simulink model "Appl_DrMemory_CtrlModel"  (R2018b)
settings: configuration reference "CodeConfig_10_ms" (kept outside this file)
undefined symbols (not defined in the file): CAL_DrMem_100MS, CAL_DrMem_90MS, D_DRMEM_SPEED_5, D_ToleranceDistance, FALSE, TRUE
libraries: DareLib x92, simulink x1
(part 1 of 3)
settings Model: Creator=Administrator  LastModifiedBy=Administrator
settings ConfigSetRef: SourceLocation=Base Workspace

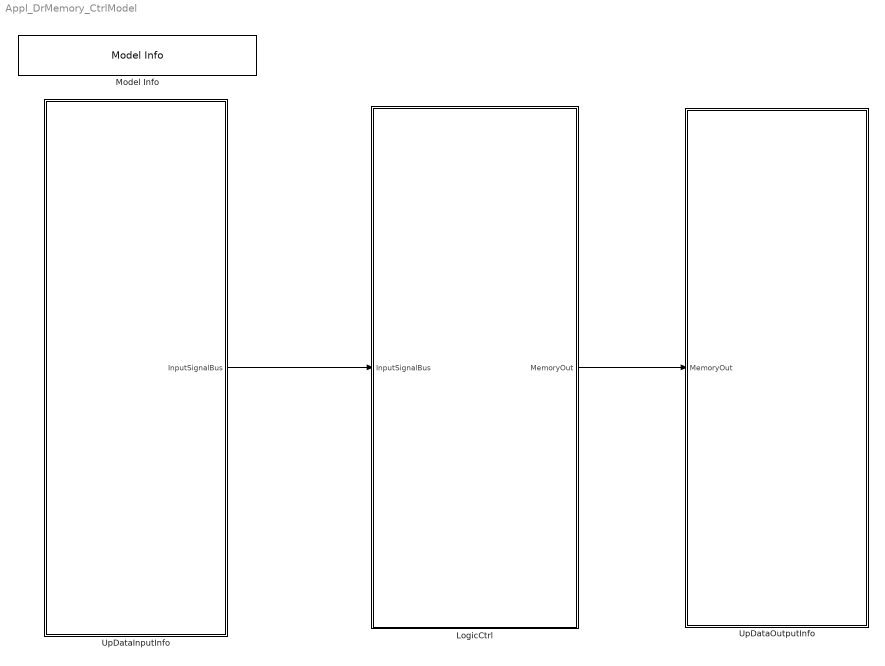
== system Appl_DrMemory_CtrlModel ==
  LogicCtrl : Subsystem  Priority=2  TreatAsAtomicUnit=on
      settings: RTWSystemCode=Nonreusable function  RTWFcnNameOpts=Use subsystem name
  Model Info : simulink/Model-Wide Utilities/Model Info  Frame=on  DisplayStringWithTags=Version：%<ModelVersion>  HorizontalTextAlignment=Center  LeftAlignmentValue=0.5
  UpDataInputInfo : Subsystem  Priority=1  TreatAsAtomicUnit=on
      settings: RTWSystemCode=Nonreusable function  RTWFcnNameOpts=Use subsystem name
  UpDataOutputInfo : Subsystem  Priority=3  TreatAsAtomicUnit=on
      settings: RTWSystemCode=Nonreusable function  RTWFcnNameOpts=Use subsystem name
  wires:
  LogicCtrl/1(MemoryOut) -> UpDataOutputInfo/1(MemoryOut)
  UpDataInputInfo/1(InputSignalBus) -> LogicCtrl/1(InputSignalBus)

== system Appl_DrMemory_CtrlModel/LogicCtrl ==
  InputSignalBus : Inport
  Bus Selector : BusSelector  OutputSignals=SpeedLessThan5_Flag,SeatMemBtn,CallMem,MemorySetPrecondition,MemoryRemindPrecondition,Rte_SignalBus.DrMem_HeightHallPosi,Rte_SignalBus.DrMem_LengthHallPosi,Rte_SignalBus.DrMem_BackHallPosi,Rte_SignalBus.DrMem_FrontHallPosi,Rte_SignalBus.DrMem_HeightAutoRunFlag,Rte_SignalBus.DrMem_LengthAutoRunFlag,Rte_SignalBus.DrMem_BackAutoRunFlag,Rte_SignalBus.DrMem_FrontAutoRunFlag,Rte_SignalBus.DrMem_AdjustEnable,Rte_SignalBus.DrMem_FLSeatPosMsg,Rte_SignalBus.DrMem_CurrentMoveType,Rte_SignalBus.DrMem_GetRecoverDefaultFlag,Rte_SignalBus.DrMem_HeightLockFault,Rte_SignalBus.DrMem_LengthLockFault,Rte_SignalBus.DrMem_BackLockFault,Rte_SignalBus.DrMem_FrontLockFault
  LocalAdjustCtrl : Subsystem  Description=加热逻辑处理
      settings: AttributesFormatString=%<Description>
  MainVent_OutputLvlSts : BusCreator  Inputs=14
  MemoryOut : Outport
  wires:
  InputSignalBus/1 -> Bus Selector/1  "InputSignalBus"
  MainVent_OutputLvlSts/1 -> MemoryOut/1  "MemoryOut"
  Bus Selector/2 -> LocalAdjustCtrl/1(SeatMemBtn)  "<SeatMemBtn>"
  Bus Selector/3 -> LocalAdjustCtrl/2(CallMem)  "<CallMem>"
  Bus Selector/4 -> LocalAdjustCtrl/3(MemorySetPrecondition)  "<MemorySetPrecondition>"
  Bus Selector/5 -> LocalAdjustCtrl/4(MemoryRemindPrecondition)  "<MemoryRemindPrecondition>"
  Bus Selector/6 -> LocalAdjustCtrl/5(DrMem_HeightHallPosi)  "<DrMem_HeightHallPosi>"
  Bus Selector/7 -> LocalAdjustCtrl/6(DrMem_LengthHallPosi)  "<DrMem_LengthHallPosi>"
  Bus Selector/8 -> LocalAdjustCtrl/7(DrMem_BackHallPosi)  "<DrMem_BackHallPosi>"
  Bus Selector/9 -> LocalAdjustCtrl/8(DrMem_FrontHallPosi)  "<DrMem_FrontHallPosi>"
  Bus Selector/10 -> LocalAdjustCtrl/9(DrMem_HeightAutoRunFlag)  "<DrMem_HeightAutoRunFlag>"
  Bus Selector/11 -> LocalAdjustCtrl/10(DrMem_LengthAutoRunFlag)  "<DrMem_LengthAutoRunFlag>"
  Bus Selector/12 -> LocalAdjustCtrl/11(DrMem_BackAutoRunFlag)  "<DrMem_BackAutoRunFlag>"
  Bus Selector/13 -> LocalAdjustCtrl/12(DrMem_FrontAutoRunFlag)  "<DrMem_FrontAutoRunFlag>"
  Bus Selector/14 -> LocalAdjustCtrl/13(DrMem_AdjustEnable)  "<DrMem_AdjustEnable>"
  Bus Selector/15 -> LocalAdjustCtrl/14(DrMem_FLSeatPosMsg)  "<DrMem_FLSeatPosMsg>"
  Bus Selector/16 -> LocalAdjustCtrl/15(DrMem_CurrentMoveType)  "<DrMem_CurrentMoveType>"
  Bus Selector/17 -> LocalAdjustCtrl/16(DrMem_GetRecoverDefaultFlag)  "<DrMem_GetRecoverDefaultFlag>"
  Bus Selector/18 -> LocalAdjustCtrl/17(DrMem_HeightLockFault)  "<DrMem_HeightLockFault>"
  Bus Selector/19 -> LocalAdjustCtrl/18(DrMem_LengthLockFault)  "<DrMem_LengthLockFault>"
  Bus Selector/20 -> LocalAdjustCtrl/19(DrMem_BackLockFault)  "<DrMem_BackLockFault>"
  Bus Selector/21 -> LocalAdjustCtrl/20(DrMem_FrontLockFault)  "<DrMem_FrontLockFault>"
  LocalAdjustCtrl/1(FLSeatMemSetSts) -> MainVent_OutputLvlSts/2
  LocalAdjustCtrl/2(MemSetStopReason) -> MainVent_OutputLvlSts/3
  LocalAdjustCtrl/3(FLSeatPosMsg) -> MainVent_OutputLvlSts/4
  LocalAdjustCtrl/4(SeatMemoryValidReq) -> MainVent_OutputLvlSts/5
  LocalAdjustCtrl/5(SeatHeightPosiReq) -> MainVent_OutputLvlSts/6
  LocalAdjustCtrl/6(SeatLengthPosiReq) -> MainVent_OutputLvlSts/7
  LocalAdjustCtrl/7(SeatBackPosiReq) -> MainVent_OutputLvlSts/8
  LocalAdjustCtrl/8(SeatFrontPosiReq) -> MainVent_OutputLvlSts/9
  LocalAdjustCtrl/9(MemCallStopReason) -> MainVent_OutputLvlSts/10
  LocalAdjustCtrl/10(SeatMem1StsFb) -> MainVent_OutputLvlSts/11
  LocalAdjustCtrl/11(SeatMem2StsFb) -> MainVent_OutputLvlSts/12
  LocalAdjustCtrl/12(SeatMem3StsFb) -> MainVent_OutputLvlSts/13
  LocalAdjustCtrl/13(PreMemRemindStop) -> MainVent_OutputLvlSts/14
  Bus Selector/1 -> MainVent_OutputLvlSts/1  "<SpeedLessThan5_Flag>"

== system Appl_DrMemory_CtrlModel/UpDataInputInfo ==
  InputSignalProcess : Subsystem  Description=数据处理
      settings: AttributesFormatString=%<Description>  RTWSystemCode=Nonreusable function  RTWFcnNameOpts=Use subsystem name
  RTE : Subsystem  Description=接口自动生成  TreatAsAtomicUnit=on
      settings: AttributesFormatString=%<Description>  RTWSystemCode=Nonreusable function  RTWFcnNameOpts=Use subsystem name
  InputSignalBus : Outport
  wires:
  RTE/1(RTE_Signal) -> InputSignalProcess/1(Rte_SignalBus)
  InputSignalProcess/1(InputSignalBus) -> InputSignalBus/1

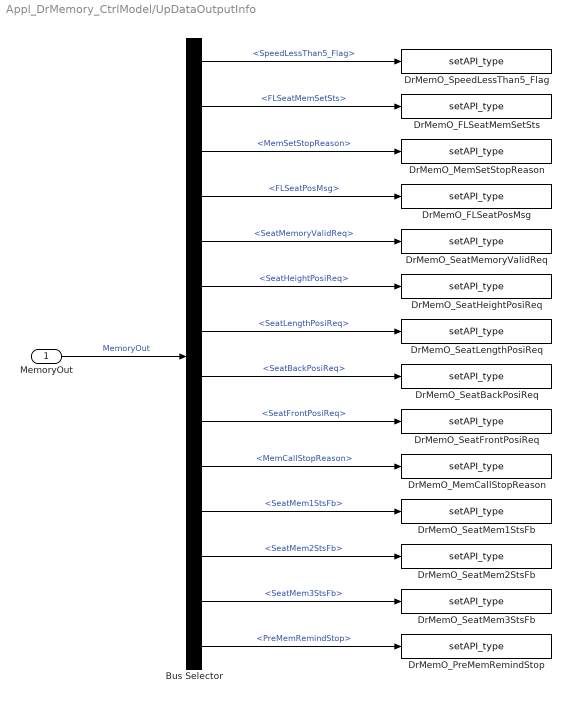
== system Appl_DrMemory_CtrlModel/UpDataOutputInfo ==
  MemoryOut : Inport
  Bus Selector : BusSelector  OutputSignals=SpeedLessThan5_Flag,FLSeatMemSetSts,MemSetStopReason,FLSeatPosMsg,SeatMemoryValidReq,SeatHeightPosiReq,SeatLengthPosiReq,SeatBackPosiReq,SeatFrontPosiReq,MemCallStopReason,SeatMem1StsFb,SeatMem2StsFb,SeatMem3StsFb,PreMemRemindStop
  DrMemO_FLSeatMemSetSts : DareLib/Dare/setAPI_type  g_funcname=CanTx_0x3B2_DSM_FLSeatMemStsAndMsg  g_param=""  g_type=uint8  g_enum=enMemSetFb  g_size=-1
      settings: AttributesFormatString=%<g_funcname>  SourceProductName=Dare Library
  DrMemO_FLSeatPosMsg : DareLib/Dare/setAPI_type  g_funcname=CanTx_0x3B2_DSM_FLSeatPosMsg  g_param=""  g_type=uint8  g_size=-1
      settings: AttributesFormatString=%<g_funcname>  SourceProductName=Dare Library
  DrMemO_MemCallStopReason : DareLib/Dare/setAPI_type  g_funcname=Rte_SetVfb_MemCallStopReason  g_param=""  g_type=uint8  g_enum=enMemStopCause  g_size=-1
      settings: AttributesFormatString=%<g_funcname>  SourceProductName=Dare Library
  DrMemO_MemSetStopReason : DareLib/Dare/setAPI_type  g_funcname=Rte_SetVfb_MemSetStopReason  g_param=""  g_type=uint8  g_enum=enMemStopCause  g_size=-1
      settings: AttributesFormatString=%<g_funcname>  SourceProductName=Dare Library
  DrMemO_PreMemRemindStop : DareLib/Dare/setAPI_type  g_funcname=Rte_SetVfb_PreMemRemindStop  g_param=""  g_type=uint8  g_enum=enMemStopCause  g_size=-1
      settings: AttributesFormatString=%<g_funcname>  SourceProductName=Dare Library
  DrMemO_SeatBackPosiReq : DareLib/Dare/setAPI_type  g_funcname=Rte_SetVfb_DrMemBackReqPosi  g_param=""  g_type=uint16  g_size=-1
      settings: AttributesFormatString=%<g_funcname>  SourceProductName=Dare Library
  DrMemO_SeatFrontPosiReq : DareLib/Dare/setAPI_type  g_funcname=Rte_SetVfb_DrMemFrontReqPosi  g_param=""  g_type=uint16  g_size=-1
      settings: AttributesFormatString=%<g_funcname>  SourceProductName=Dare Library
  DrMemO_SeatHeightPosiReq : DareLib/Dare/setAPI_type  g_funcname=Rte_SetVfb_DrMemHeightReqPosi  g_param=""  g_type=uint16  g_size=-1
      settings: AttributesFormatString=%<g_funcname>  SourceProductName=Dare Library
  DrMemO_SeatLengthPosiReq : DareLib/Dare/setAPI_type  g_funcname=Rte_SetVfb_DrMemLengthReqPosi  g_param=""  g_type=uint16  g_size=-1
      settings: AttributesFormatString=%<g_funcname>  SourceProductName=Dare Library
  DrMemO_SeatMem1StsFb : DareLib/Dare/setAPI_type  g_funcname=CanTx_0x3B2_DSM1_FLSeatMem1Sts  g_param=""  g_type=uint8  g_enum=enMemCallFb  g_size=-1
      settings: AttributesFormatString=%<g_funcname>  SourceProductName=Dare Library
  DrMemO_SeatMem2StsFb : DareLib/Dare/setAPI_type  g_funcname=CanTx_0x3B2_DSM2_FLSeatMem2Sts  g_param=""  g_type=uint8  g_enum=enMemCallFb  g_size=-1
      settings: AttributesFormatString=%<g_funcname>  SourceProductName=Dare Library
  DrMemO_SeatMem3StsFb : DareLib/Dare/setAPI_type  g_funcname=CanTx_0x3B2_DSM3_FLSeatMem3Sts  g_param=""  g_type=uint8  g_enum=enMemCallFb  g_size=-1
      settings: AttributesFormatString=%<g_funcname>  SourceProductName=Dare Library
  DrMemO_SeatMemoryValidReq : DareLib/Dare/setAPI_type  g_funcname=Rte_SetVfb_SeatMemoryValidReq  g_param=""  g_type=uint8  g_size=-1
      settings: AttributesFormatString=%<g_funcname>  SourceProductName=Dare Library
  DrMemO_SpeedLessThan5_Flag : DareLib/Dare/setAPI_type  g_funcname=Rte_SetVfb_SpeedLessThan5_Flag  g_param=""  g_type=uint8  g_size=-1
      settings: AttributesFormatString=%<g_funcname>  SourceProductName=Dare Library
  wires:
  MemoryOut/1 -> Bus Selector/1  "MemoryOut"
  Bus Selector/1 -> DrMemO_SpeedLessThan5_Flag/1  "<SpeedLessThan5_Flag>"
  Bus Selector/2 -> DrMemO_FLSeatMemSetSts/1  "<FLSeatMemSetSts>"
  Bus Selector/3 -> DrMemO_MemSetStopReason/1  "<MemSetStopReason>"
  Bus Selector/4 -> DrMemO_FLSeatPosMsg/1  "<FLSeatPosMsg>"
  Bus Selector/5 -> DrMemO_SeatMemoryValidReq/1  "<SeatMemoryValidReq>"
  Bus Selector/6 -> DrMemO_SeatHeightPosiReq/1  "<SeatHeightPosiReq>"
  Bus Selector/7 -> DrMemO_SeatLengthPosiReq/1  "<SeatLengthPosiReq>"
  Bus Selector/8 -> DrMemO_SeatBackPosiReq/1  "<SeatBackPosiReq>"
  Bus Selector/9 -> DrMemO_SeatFrontPosiReq/1  "<SeatFrontPosiReq>"
  Bus Selector/10 -> DrMemO_MemCallStopReason/1  "<MemCallStopReason>"
  Bus Selector/11 -> DrMemO_SeatMem1StsFb/1  "<SeatMem1StsFb>"
  Bus Selector/12 -> DrMemO_SeatMem2StsFb/1  "<SeatMem2StsFb>"
  Bus Selector/13 -> DrMemO_SeatMem3StsFb/1  "<SeatMem3StsFb>"
  Bus Selector/14 -> DrMemO_PreMemRemindStop/1  "<PreMemRemindStop>"

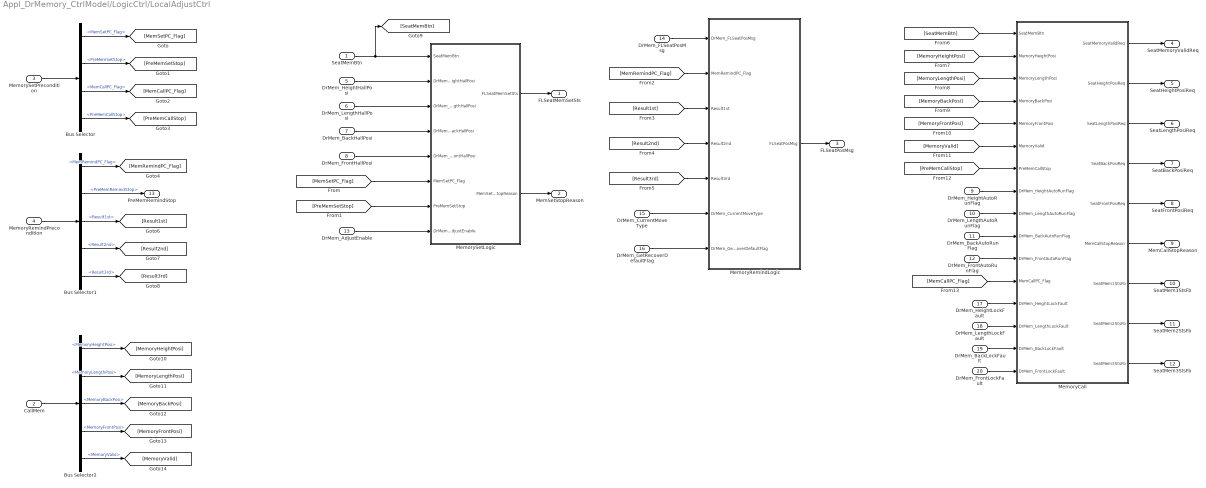
== system Appl_DrMemory_CtrlModel/LogicCtrl/LocalAdjustCtrl ==
  SeatMemBtn : Inport
  CallMem : Inport  Port=2
  MemorySetPrecondition : Inport  Port=3
  MemoryRemindPrecondition : Inport  Port=4
  DrMem_HeightHallPosi : Inport  Port=5
  DrMem_LengthHallPosi : Inport  Port=6
  DrMem_BackHallPosi : Inport  Port=7
  DrMem_FrontHallPosi : Inport  Port=8
  DrMem_HeightAutoRunFlag : Inport  Port=9
  DrMem_LengthAutoRunFlag : Inport  Port=10
  DrMem_BackAutoRunFlag : Inport  Port=11
  DrMem_FrontAutoRunFlag : Inport  Port=12
  DrMem_AdjustEnable : Inport  Port=13
  DrMem_FLSeatPosMsg : Inport  Port=14
  DrMem_CurrentMoveType : Inport  Port=15
  DrMem_GetRecoverDefaultFlag : Inport  Port=16
  DrMem_HeightLockFault : Inport  Port=17
  DrMem_LengthLockFault : Inport  Port=18
  DrMem_BackLockFault : Inport  Port=19
  DrMem_FrontLockFault : Inport  Port=20
  Bus Selector : BusSelector  OutputSignals=MemSetPC_Flag,PreMemSetStop,MemCallPC_Flag,PreMemCallStop
  Bus Selector1 : BusSelector  OutputSignals=MemRemindPC_Flag,PreMemRemindStop,Result1st,Result2nd,Result3rd
  Bus Selector2 : BusSelector  OutputSignals=MemoryHeightPosi,MemoryLengthPosi,MemoryBackPosi,MemoryFrontPosi,MemoryValid
  MemoryCall : Stateflow chart  TreatAsAtomicUnit=on
  MemoryRemindLogic : Stateflow chart  TreatAsAtomicUnit=on
  MemorySetLogic : Stateflow chart  TreatAsAtomicUnit=on
  FLSeatMemSetSts : Outport
  MemSetStopReason : Outport  Port=2
  FLSeatPosMsg : Outport  Port=3
  SeatMemoryValidReq : Outport  Port=4
  SeatHeightPosiReq : Outport  Port=5
  SeatLengthPosiReq : Outport  Port=6
  SeatBackPosiReq : Outport  Port=7
  SeatFrontPosiReq : Outport  Port=8
  MemCallStopReason : Outport  Port=9
  SeatMem1StsFb : Outport  Port=10
  SeatMem2StsFb : Outport  Port=11
  SeatMem3StsFb : Outport  Port=12
  PreMemRemindStop : Outport  Port=13
  wires:
  SeatMemBtn/1 -> [SeatMemBtn], MemorySetLogic/1(SeatMemBtn)
  DrMem_HeightHallPosi/1 -> MemorySetLogic/2(DrMem_HeightHallPosi)
  DrMem_LengthHallPosi/1 -> MemorySetLogic/3(DrMem_LengthHallPosi)
  DrMem_BackHallPosi/1 -> MemorySetLogic/4(DrMem_BackHallPosi)
  DrMem_FrontHallPosi/1 -> MemorySetLogic/5(DrMem_FrontHallPosi)
  MemorySetPrecondition/1 -> Bus Selector/1
  Bus Selector/1 -> [MemSetPC_Flag]  "<MemSetPC_Flag>"
  Bus Selector/2 -> [PreMemSetStop]  "<PreMemSetStop>"
  Bus Selector/3 -> [MemCallPC_Flag]  "<MemCallPC_Flag>"
  Bus Selector/4 -> [PreMemCallStop]  "<PreMemCallStop>"
  [MemSetPC_Flag] -> MemorySetLogic/6(MemSetPC_Flag)
  [PreMemSetStop] -> MemorySetLogic/7(PreMemSetStop)
  DrMem_AdjustEnable/1 -> MemorySetLogic/8(DrMem_AdjustEnable)
  MemoryRemindPrecondition/1 -> Bus Selector1/1
  Bus Selector1/4 -> [Result2nd]  "<Result2nd>"
  Bus Selector1/3 -> [Result1st]  "<Result1st>"
  Bus Selector1/5 -> [Result3rd]  "<Result3rd>"
  Bus Selector1/1 -> [MemRemindPC_Flag]  "<MemRemindPC_Flag>"
  DrMem_FLSeatPosMsg/1 -> MemoryRemindLogic/1(DrMem_FLSeatPosMsg)
  [MemRemindPC_Flag] -> MemoryRemindLogic/2(MemRemindPC_Flag)
  [Result1st] -> MemoryRemindLogic/3(Result1st)
  [Result2nd] -> MemoryRemindLogic/4(Result2nd)
  [Result3rd] -> MemoryRemindLogic/5(Result3rd)
  DrMem_CurrentMoveType/1 -> MemoryRemindLogic/6(DrMem_CurrentMoveType)
  DrMem_GetRecoverDefaultFlag/1 -> MemoryRemindLogic/7(DrMem_GetRecoverDefaultFlag)
  CallMem/1 -> Bus Selector2/1
  Bus Selector2/1 -> [MemoryHeightPosi]  "<MemoryHeightPosi>"
  Bus Selector2/2 -> [MemoryLengthPosi]  "<MemoryLengthPosi>"
  Bus Selector2/3 -> [MemoryBackPosi]  "<MemoryBackPosi>"
  Bus Selector2/4 -> [MemoryFrontPosi]  "<MemoryFrontPosi>"
  Bus Selector2/5 -> [MemoryValid]  "<MemoryValid>"
  [SeatMemBtn] -> MemoryCall/1(SeatMemBtn)
  [MemoryHeightPosi] -> MemoryCall/2(MemoryHeightPosi)
  [MemoryLengthPosi] -> MemoryCall/3(MemoryLengthPosi)
  [MemoryBackPosi] -> MemoryCall/4(MemoryBackPosi)
  [MemoryFrontPosi] -> MemoryCall/5(MemoryFrontPosi)
  [MemoryValid] -> MemoryCall/6(MemoryValid)
  [PreMemCallStop] -> MemoryCall/7(PreMemCallStop)
  DrMem_HeightAutoRunFlag/1 -> MemoryCall/8(DrMem_HeightAutoRunFlag)
  DrMem_LengthAutoRunFlag/1 -> MemoryCall/9(DrMem_LengthAutoRunFlag)
  DrMem_BackAutoRunFlag/1 -> MemoryCall/10(DrMem_BackAutoRunFlag)
  DrMem_FrontAutoRunFlag/1 -> MemoryCall/11(DrMem_FrontAutoRunFlag)
  [MemCallPC_Flag] -> MemoryCall/12(MemCallPC_Flag)
  DrMem_FrontLockFault/1 -> MemoryCall/16(DrMem_FrontLockFault)
  DrMem_BackLockFault/1 -> MemoryCall/15(DrMem_BackLockFault)
  DrMem_LengthLockFault/1 -> MemoryCall/14(DrMem_LengthLockFault)
  DrMem_HeightLockFault/1 -> MemoryCall/13(DrMem_HeightLockFault)
  MemorySetLogic/1(FLSeatMemSetSts) -> FLSeatMemSetSts/1
  MemorySetLogic/2(MemSetStopReason) -> MemSetStopReason/1
  MemoryRemindLogic/1(FLSeatPosMsg) -> FLSeatPosMsg/1
  MemoryCall/1(SeatMemoryValidReq) -> SeatMemoryValidReq/1
  MemoryCall/2(SeatHeightPosiReq) -> SeatHeightPosiReq/1
  MemoryCall/3(SeatLengthPosiReq) -> SeatLengthPosiReq/1
  MemoryCall/4(SeatBackPosiReq) -> SeatBackPosiReq/1
  MemoryCall/5(SeatFrontPosiReq) -> SeatFrontPosiReq/1
  MemoryCall/6(MemCallStopReason) -> MemCallStopReason/1
  MemoryCall/7(SeatMem1StsFb) -> SeatMem1StsFb/1
  MemoryCall/8(SeatMem2StsFb) -> SeatMem2StsFb/1
  MemoryCall/9(SeatMem3StsFb) -> SeatMem3StsFb/1
  Bus Selector1/2 -> PreMemRemindStop/1  "<PreMemRemindStop>"

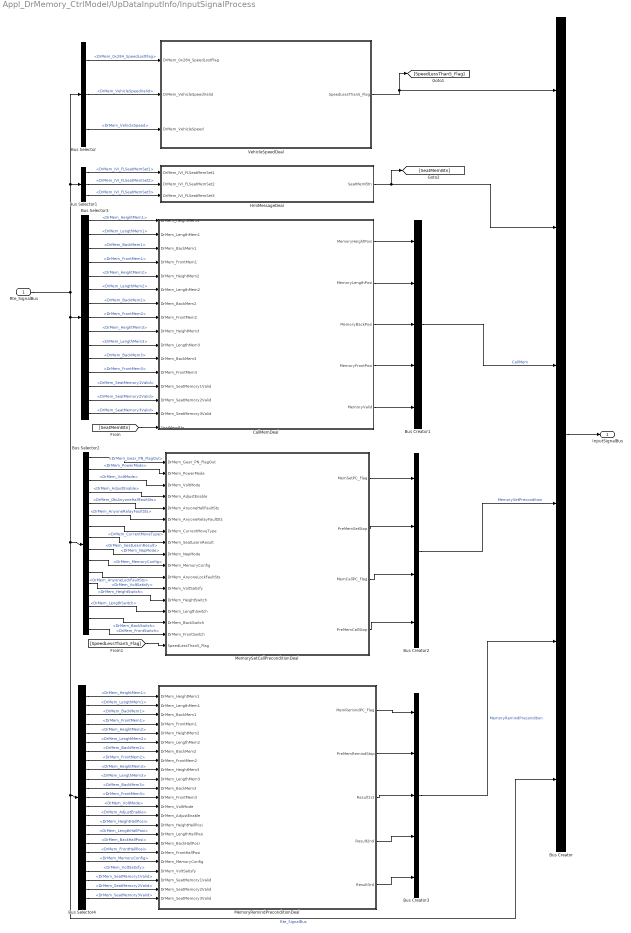
== system Appl_DrMemory_CtrlModel/UpDataInputInfo/InputSignalProcess ==
  Rte_SignalBus : Inport
  Bus Creator : BusCreator  Inputs=6
  Bus Creator1 : BusCreator  Inputs=5
  Bus Creator2 : BusCreator  Inputs=4
  Bus Creator3 : BusCreator  Inputs=5
  Bus Selector : BusSelector  OutputSignals=DrMem_0x284_SpeedLostFlag,DrMem_VehicleSpeedValid,DrMem_VehicleSpeed
  Bus Selector1 : BusSelector  OutputSignals=DrMem_IVI_FLSeatMemSet1,DrMem_IVI_FLSeatMemSet2,DrMem_IVI_FLSeatMemSet3
  Bus Selector2 : BusSelector  OutputSignals=DrMem_Gear_PN_FlagOut,DrMem_PowerMode,DrMem_VoltMode,DrMem_AdjustEnable,DrMem_DtcAnyoneHallFaultSts,DrMem_AnyoneRelayFaultSts,DrMem_CurrentMoveType,DrMem_SeatLearnResult,DrMem_NapMode,DrMem_MemoryConfig,DrMem_AnyoneLockFaultSts,DrMem_VoltSatisfy,DrMem_HeightSwitch,DrMem_LengthSwitch,DrMem_BackSwitch,DrMem_FrontSwitch
  Bus Selector3 : BusSelector  OutputSignals=DrMem_HeightMem1,DrMem_LengthMem1,DrMem_BackMem1,DrMem_FrontMem1,DrMem_HeightMem2,DrMem_LengthMem2,DrMem_BackMem2,DrMem_FrontMem2,DrMem_HeightMem3,DrMem_LengthMem3,DrMem_BackMem3,DrMem_FrontMem3,DrMem_SeatMemory1Valid,DrMem_SeatMemory2Valid,DrMem_SeatMemory3Valid
  Bus Selector4 : BusSelector  OutputSignals=DrMem_HeightMem1,DrMem_LengthMem1,DrMem_BackMem1,DrMem_FrontMem1,DrMem_HeightMem2,DrMem_LengthMem2,DrMem_BackMem2,DrMem_FrontMem2,DrMem_HeightMem3,DrMem_LengthMem3,DrMem_BackMem3,DrMem_FrontMem3,DrMem_VoltMode,DrMem_AdjustEnable,DrMem_HeightHallPosi,DrMem_LengthHallPosi,DrMem_BackHallPosi,DrMem_FrontHallPosi,DrMem_MemoryConfig,DrMem_VoltSatisfy,DrMem_SeatMemory1Valid,DrMem_SeatMemory2Valid,DrMem_SeatMemory3Valid
  CallMemDeal : Subsystem  Description=记忆调用位置处理
      settings: AttributesFormatString=%<Description>
  HmiMessageDeal : Subsystem  Description=记忆报文处理
      settings: AttributesFormatString=%<Description>
  MemoryRemindPreconditionDeal : Subsystem  Description=记忆提示前置条件处理
      settings: AttributesFormatString=%<Description>
  MemorySetCallPreconditionDeal : Subsystem  Description=记忆设置与调用前置条件处理
      settings: AttributesFormatString=%<Description>
  VehicleSpeedDeal : Subsystem  Description=车速报文处理
      settings: AttributesFormatString=%<Description>
  InputSignalBus : Outport
  wires:
  Bus Creator/1 -> InputSignalBus/1
  Rte_SignalBus/1 -> Bus Creator/6, Bus Selector4/1, Bus Selector2/1, Bus Selector3/1, Bus Selector/1, Bus Selector1/1  "Rte_SignalBus"
  VehicleSpeedDeal/1("SpeedLessThan5_Flag ") -> [SpeedLessThan5_Flag], Bus Creator/1
  HmiMessageDeal/1(SeatMemBtn) -> [SeatMemBtn], Bus Creator/2
  Bus Selector/1 -> VehicleSpeedDeal/1(DrMem_0x284_SpeedLostFlag)  "<DrMem_0x284_SpeedLostFlag>"
  Bus Selector/2 -> VehicleSpeedDeal/2(DrMem_VehicleSpeedValid)  "<DrMem_VehicleSpeedValid>"
  Bus Selector/3 -> VehicleSpeedDeal/3(DrMem_VehicleSpeed)  "<DrMem_VehicleSpeed>"
  Bus Selector1/1 -> HmiMessageDeal/1(DrMem_IVI_FLSeatMemSet1)  "<DrMem_IVI_FLSeatMemSet1>"
  Bus Selector1/2 -> HmiMessageDeal/2(DrMem_IVI_FLSeatMemSet2)  "<DrMem_IVI_FLSeatMemSet2>"
  Bus Selector1/3 -> HmiMessageDeal/3(DrMem_IVI_FLSeatMemSet3)  "<DrMem_IVI_FLSeatMemSet3>"
  Bus Selector3/1 -> CallMemDeal/1(DrMem_HeightMem1)  "<DrMem_HeightMem1>"
  Bus Selector3/2 -> CallMemDeal/2(DrMem_LengthMem1)  "<DrMem_LengthMem1>"
  Bus Selector3/3 -> CallMemDeal/3(DrMem_BackMem1)  "<DrMem_BackMem1>"
  Bus Selector3/4 -> CallMemDeal/4(DrMem_FrontMem1)  "<DrMem_FrontMem1>"
  Bus Selector3/5 -> CallMemDeal/5(DrMem_HeightMem2)  "<DrMem_HeightMem2>"
  Bus Selector3/6 -> CallMemDeal/6(DrMem_LengthMem2)  "<DrMem_LengthMem2>"
  Bus Selector3/7 -> CallMemDeal/7(DrMem_BackMem2)  "<DrMem_BackMem2>"
  Bus Selector3/8 -> CallMemDeal/8(DrMem_FrontMem2)  "<DrMem_FrontMem2>"
  Bus Selector3/9 -> CallMemDeal/9(DrMem_HeightMem3)  "<DrMem_HeightMem3>"
  Bus Selector3/10 -> CallMemDeal/10(DrMem_LengthMem3)  "<DrMem_LengthMem3>"
  Bus Selector3/11 -> CallMemDeal/11(DrMem_BackMem3)  "<DrMem_BackMem3>"
  Bus Selector3/12 -> CallMemDeal/12(DrMem_FrontMem3)  "<DrMem_FrontMem3>"
  [SeatMemBtn] -> CallMemDeal/16(SeatMemBtn)
  CallMemDeal/1(MemoryHeightPosi) -> Bus Creator1/1
  CallMemDeal/2(MemoryLengthPosi) -> Bus Creator1/2
  CallMemDeal/3(MemoryBackPosi) -> Bus Creator1/3
  CallMemDeal/4(MemoryFrontPosi) -> Bus Creator1/4
  CallMemDeal/5(MemoryValid) -> Bus Creator1/5
  Bus Selector2/2 -> MemorySetCallPreconditionDeal/2(DrMem_PowerMode)  "<DrMem_PowerMode>"
  Bus Selector2/1 -> MemorySetCallPreconditionDeal/1(DrMem_Gear_PN_FlagOut)  "<DrMem_Gear_PN_FlagOut>"
  Bus Selector2/3 -> MemorySetCallPreconditionDeal/3(DrMem_VoltMode)  "<DrMem_VoltMode>"
  Bus Selector2/4 -> MemorySetCallPreconditionDeal/4(DrMem_AdjustEnable)  "<DrMem_AdjustEnable>"
  Bus Selector2/5 -> MemorySetCallPreconditionDeal/5(DrMem_AnyoneHallFaultSts)  "<DrMem_DtcAnyoneHallFaultSts>"
  Bus Selector2/7 -> MemorySetCallPreconditionDeal/7(DrMem_CurrentMoveType)  "<DrMem_CurrentMoveType>"
  Bus Selector2/8 -> MemorySetCallPreconditionDeal/8(DrMem_SeatLearnResult)  "<DrMem_SeatLearnResult>"
  Bus Selector2/9 -> MemorySetCallPreconditionDeal/9(DrMem_NapMode)  "<DrMem_NapMode>"
  [SpeedLessThan5_Flag] -> MemorySetCallPreconditionDeal/17(SpeedLessThan5_Flag)
  Bus Selector2/6 -> MemorySetCallPreconditionDeal/6(DrMem_AnyoneRelayFaultSts)  "<DrMem_AnyoneRelayFaultSts>"
  Bus Selector4/5 -> MemoryRemindPreconditionDeal/5(DrMem_HeightMem2)  "<DrMem_HeightMem2>"
  Bus Selector4/4 -> MemoryRemindPreconditionDeal/4(DrMem_FrontMem1)  "<DrMem_FrontMem1>"
  Bus Selector4/6 -> MemoryRemindPreconditionDeal/6(DrMem_LengthMem2)  "<DrMem_LengthMem2>"
  Bus Selector4/3 -> MemoryRemindPreconditionDeal/3(DrMem_BackMem1)  "<DrMem_BackMem1>"
  Bus Selector4/7 -> MemoryRemindPreconditionDeal/7(DrMem_BackMem2)  "<DrMem_BackMem2>"
  Bus Selector4/2 -> MemoryRemindPreconditionDeal/2(DrMem_LengthMem1)  "<DrMem_LengthMem1>"
  Bus Selector4/8 -> MemoryRemindPreconditionDeal/8(DrMem_FrontMem2)  "<DrMem_FrontMem2>"
  Bus Selector4/1 -> MemoryRemindPreconditionDeal/1(DrMem_HeightMem1)  "<DrMem_HeightMem1>"
  Bus Selector4/9 -> MemoryRemindPreconditionDeal/9(DrMem_HeightMem3)  "<DrMem_HeightMem3>"
  Bus Selector4/10 -> MemoryRemindPreconditionDeal/10(DrMem_LengthMem3)  "<DrMem_LengthMem3>"
  Bus Selector4/11 -> MemoryRemindPreconditionDeal/11(DrMem_BackMem3)  "<DrMem_BackMem3>"
  Bus Selector4/12 -> MemoryRemindPreconditionDeal/12(DrMem_FrontMem3)  "<DrMem_FrontMem3>"
  Bus Selector4/13 -> MemoryRemindPreconditionDeal/13(DrMem_VoltMode)  "<DrMem_VoltMode>"
  Bus Selector4/14 -> MemoryRemindPreconditionDeal/14(DrMem_AdjustEnable)  "<DrMem_AdjustEnable>"
  Bus Selector4/15 -> MemoryRemindPreconditionDeal/15(DrMem_HeightHallPosi)  "<DrMem_HeightHallPosi>"
  Bus Selector4/16 -> MemoryRemindPreconditionDeal/16(DrMem_LengthHallPosi)  "<DrMem_LengthHallPosi>"
  Bus Selector4/17 -> MemoryRemindPreconditionDeal/17(DrMem_BackHallPosi)  "<DrMem_BackHallPosi>"
  Bus Selector4/18 -> MemoryRemindPreconditionDeal/18(DrMem_FrontHallPosi)  "<DrMem_FrontHallPosi>"
  MemorySetCallPreconditionDeal/1(MemSetPC_Flag) -> Bus Creator2/1
  MemorySetCallPreconditionDeal/2(PreMemSetStop) -> Bus Creator2/2
  MemorySetCallPreconditionDeal/3(MemCallPC_Flag) -> Bus Creator2/3
  MemorySetCallPreconditionDeal/4(PreMemCallStop) -> Bus Creator2/4
  MemoryRemindPreconditionDeal/2(PreMemRemindStop) -> Bus Creator3/2
  MemoryRemindPreconditionDeal/1(MemRemindPC_Flag) -> Bus Creator3/1
  MemoryRemindPreconditionDeal/3(Result1st) -> Bus Creator3/3
  MemoryRemindPreconditionDeal/4(Result2nd) -> Bus Creator3/4
  MemoryRemindPreconditionDeal/5(Result3rd) -> Bus Creator3/5
  Bus Creator1/1 -> Bus Creator/3  "CallMem"
  Bus Creator2/1 -> Bus Creator/4  "MemorySetPrecondition"
  Bus Creator3/1 -> Bus Creator/5  "MemoryRemindPrecondition"
  Bus Selector3/13 -> CallMemDeal/13(DrMem_SeatMemory1Valid)  "<DrMem_SeatMemory1Valid>"
  Bus Selector3/14 -> CallMemDeal/14(DrMem_SeatMemory2Valid)  "<DrMem_SeatMemory2Valid>"
  Bus Selector3/15 -> CallMemDeal/15(DrMem_SeatMemory3Valid)  "<DrMem_SeatMemory3Valid>"
  Bus Selector2/10 -> MemorySetCallPreconditionDeal/10(DrMem_MemoryConfig)  "<DrMem_MemoryConfig>"
  Bus Selector4/19 -> MemoryRemindPreconditionDeal/19(DrMem_MemoryConfig)  "<DrMem_MemoryConfig>"
  Bus Selector2/11 -> MemorySetCallPreconditionDeal/11(DrMem_AnyoneLockFaultSts)  "<DrMem_AnyoneLockFaultSts>"
  Bus Selector2/12 -> MemorySetCallPreconditionDeal/12(DrMem_VoltSatisfy)  "<DrMem_VoltSatisfy>"
  Bus Selector4/20 -> MemoryRemindPreconditionDeal/20(DrMem_VoltSatisfy)  "<DrMem_VoltSatisfy>"
  Bus Selector4/21 -> MemoryRemindPreconditionDeal/21(DrMem_SeatMemory1Valid)  "<DrMem_SeatMemory1Valid>"
  Bus Selector4/22 -> MemoryRemindPreconditionDeal/22(DrMem_SeatMemory2Valid)  "<DrMem_SeatMemory2Valid>"
  Bus Selector4/23 -> MemoryRemindPreconditionDeal/23(DrMem_SeatMemory3Valid)  "<DrMem_SeatMemory3Valid>"
  Bus Selector2/13 -> MemorySetCallPreconditionDeal/13(DrMem_HeightSwitch)  "<DrMem_HeightSwitch>"
  Bus Selector2/14 -> MemorySetCallPreconditionDeal/14(DrMem_LengthSwitch)  "<DrMem_LengthSwitch>"
  Bus Selector2/15 -> MemorySetCallPreconditionDeal/15(DrMem_BackSwitch)  "<DrMem_BackSwitch>"
  Bus Selector2/16 -> MemorySetCallPreconditionDeal/16(DrMem_FrontSwitch)  "<DrMem_FrontSwitch>"

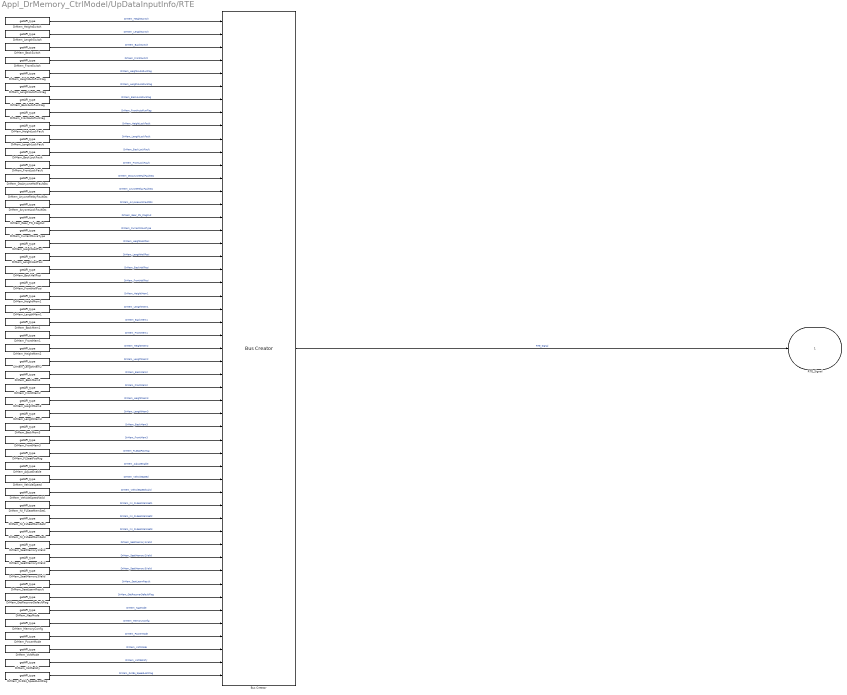
== system Appl_DrMemory_CtrlModel/UpDataInputInfo/RTE ==
  Bus Creator : BusCreator  Inputs=51
  DrMem_0x284_SpeedLostFlag : DareLib/Dare/getAPI_type  g_funcname=Ecual_GetCanMsgLostFlag  g_param=eRXINDEX_0x284  g_type=uint8  g_size=-1
      settings: AttributesFormatString=%<g_funcname>  SourceProductName=Dare Library
  DrMem_AdjustEnable : DareLib/Dare/getAPI_type  g_funcname=Srvl_GetMemIndexDataU8  g_param=EN_MemIndex_DrAdjustConfig  g_type=uint8  g_size=-1
      settings: AttributesFormatString=%<g_funcname>  SourceProductName=Dare Library
  DrMem_AnyoneLockFaultSts : DareLib/Dare/getAPI_type  g_funcname=Rte_GetVfb_DrAnyoneStallErr  g_param=""  g_type=uint8  g_size=-1
      settings: AttributesFormatString=%<g_funcname>  SourceProductName=Dare Library
  DrMem_AnyoneRelayFaultSts : DareLib/Dare/getAPI_type  g_funcname=Rte_GetVfb_DrAnyoneRelayAdheErr  g_param=""  g_type=uint8  g_enum=enSeatMotorRunType  g_size=-1
      settings: AttributesFormatString=%<g_funcname>  SourceProductName=Dare Library
  DrMem_BackAutoRunFlag : DareLib/Dare/getAPI_type  g_funcname=Rte_GetVfb_DrBackAutoRunFlag  g_param=""  g_type=uint8  g_enum=enSeatAutoRunSts  g_size=-1
      settings: AttributesFormatString=%<g_funcname>  SourceProductName=Dare Library
  DrMem_BackHallPosi : DareLib/Dare/getAPI_type  g_funcname=Cdd_GetCurrentHallCnt  g_param=EN_DriverBack  g_type=uint16  g_size=-1
      settings: AttributesFormatString=%<g_funcname>  SourceProductName=Dare Library
  DrMem_BackLockFault : DareLib/Dare/getAPI_type  g_funcname=Rte_GetVfb_DrBackStallErr  g_param=""  g_type=uint8  g_size=-1
      settings: AttributesFormatString=%<g_funcname>  SourceProductName=Dare Library
  DrMem_BackMem1 : DareLib/Dare/getAPI_type  g_funcname=Srvl_GetMemIndexDataU16  g_param=EN_MemIndex_DrMem1_Back  g_type=uint16  g_size=-1
      settings: AttributesFormatString=%<g_funcname>  SourceProductName=Dare Library
  DrMem_BackMem2 : DareLib/Dare/getAPI_type  g_funcname=Srvl_GetMemIndexDataU16  g_param=EN_MemIndex_DrMem2_Back  g_type=uint16  g_size=-1
      settings: AttributesFormatString=%<g_funcname>  SourceProductName=Dare Library
  DrMem_BackMem3 : DareLib/Dare/getAPI_type  g_funcname=Srvl_GetMemIndexDataU16  g_param=EN_MemIndex_DrMem3_Back  g_type=uint16  g_size=-1
      settings: AttributesFormatString=%<g_funcname>  SourceProductName=Dare Library
  DrMem_BackSwitch : DareLib/Dare/getAPI_type  g_funcname=Rte_GetVfb_DrBackSwitchCmd  g_param=""  g_type=uint8  g_size=-1
      settings: AttributesFormatString=%<g_funcname>  SourceProductName=Dare Library
  DrMem_CurrentMoveType : DareLib/Dare/getAPI_type  g_funcname=Rte_GetVfb_DrMoveType  g_param=""  g_type=uint8  g_size=-1
      settings: AttributesFormatString=%<g_funcname>  SourceProductName=Dare Library
  DrMem_DtcAnyoneHallFaultSts : DareLib/Dare/getAPI_type  g_funcname=Rte_GetVfb_DrAnyoneHallErr  g_param=""  g_type=uint8  g_size=-1
      settings: AttributesFormatString=%<g_funcname>  SourceProductName=Dare Library
  DrMem_FLSeatPosMsg : DareLib/Dare/getAPI_type  g_funcname=Srvl_GetMemIndexDataU8  g_param=EN_MemIndex_FLSeatPosMsg  g_type=uint8  g_size=-1
      settings: AttributesFormatString=%<g_funcname>  SourceProductName=Dare Library
  DrMem_FrontAutoRunFlag : DareLib/Dare/getAPI_type  g_funcname=Rte_GetVfb_DrFrontAutoRunFlag  g_param=""  g_type=uint8  g_enum=enSeatAutoRunSts  g_size=-1
      settings: AttributesFormatString=%<g_funcname>  SourceProductName=Dare Library
  DrMem_FrontHallPosi : DareLib/Dare/getAPI_type  g_funcname=Cdd_GetCurrentHallCnt  g_param=EN_DriverFront  g_type=uint16  g_size=-1
      settings: AttributesFormatString=%<g_funcname>  SourceProductName=Dare Library
  DrMem_FrontLockFault : DareLib/Dare/getAPI_type  g_funcname=Rte_GetVfb_DrFrontStallErr  g_param=""  g_type=uint8  g_size=-1
      settings: AttributesFormatString=%<g_funcname>  SourceProductName=Dare Library
  DrMem_FrontMem1 : DareLib/Dare/getAPI_type  g_funcname=Srvl_GetMemIndexDataU16  g_param=EN_MemIndex_DrMem1_Front  g_type=uint16  g_size=-1
      settings: AttributesFormatString=%<g_funcname>  SourceProductName=Dare Library
  DrMem_FrontMem2 : DareLib/Dare/getAPI_type  g_funcname=Srvl_GetMemIndexDataU16  g_param=EN_MemIndex_DrMem2_Front  g_type=uint16  g_size=-1
      settings: AttributesFormatString=%<g_funcname>  SourceProductName=Dare Library
  DrMem_FrontMem3 : DareLib/Dare/getAPI_type  g_funcname=Srvl_GetMemIndexDataU16  g_param=EN_MemIndex_DrMem3_Front  g_type=uint16  g_size=-1
      settings: AttributesFormatString=%<g_funcname>  SourceProductName=Dare Library
  DrMem_FrontSwitch : DareLib/Dare/getAPI_type  g_funcname=Rte_GetVfb_DrFrontSwitchCmd  g_param=""  g_type=uint8  g_size=-1
      settings: AttributesFormatString=%<g_funcname>  SourceProductName=Dare Library
  DrMem_Gear_PN_FlagOut : DareLib/Dare/getAPI_type  g_funcname=Rte_GetCAN_Gear_PN_Flag  g_param=""  g_type=uint8  g_size=-1
      settings: AttributesFormatString=%<g_funcname>  SourceProductName=Dare Library
  DrMem_GetRecoverDefaultFlag : DareLib/Dare/getAPI_type  g_funcname=GetRecoverDefaultFlag  g_param=""  g_type=uint16  g_size=-1
      settings: AttributesFormatString=%<g_funcname>  SourceProductName=Dare Library
  DrMem_HeightAutoRunFlag : DareLib/Dare/getAPI_type  g_funcname=Rte_GetVfb_DrHeightAutoRunFlag  g_param=""  g_type=uint8  g_enum=enSeatAutoRunSts  g_size=-1
      settings: AttributesFormatString=%<g_funcname>  SourceProductName=Dare Library
  DrMem_HeightHallPosi : DareLib/Dare/getAPI_type  g_funcname=Cdd_GetCurrentHallCnt  g_param=EN_DriverHeight  g_type=uint16  g_size=-1
      settings: AttributesFormatString=%<g_funcname>  SourceProductName=Dare Library
  DrMem_HeightLockFault : DareLib/Dare/getAPI_type  g_funcname=Rte_GetVfb_DrHeightStallErr  g_param=""  g_type=uint8  g_size=-1
      settings: AttributesFormatString=%<g_funcname>  SourceProductName=Dare Library
  DrMem_HeightMem1 : DareLib/Dare/getAPI_type  g_funcname=Srvl_GetMemIndexDataU16  g_param=EN_MemIndex_DrMem1_Height  g_type=uint16  g_size=-1
      settings: AttributesFormatString=%<g_funcname>  SourceProductName=Dare Library
  DrMem_HeightMem2 : DareLib/Dare/getAPI_type  g_funcname=Srvl_GetMemIndexDataU16  g_param=EN_MemIndex_DrMem2_Height  g_type=uint16  g_size=-1
      settings: AttributesFormatString=%<g_funcname>  SourceProductName=Dare Library
  DrMem_HeightMem3 : DareLib/Dare/getAPI_type  g_funcname=Srvl_GetMemIndexDataU16  g_param=EN_MemIndex_DrMem3_Height  g_type=uint16  g_size=-1
      settings: AttributesFormatString=%<g_funcname>  SourceProductName=Dare Library
  DrMem_HeightSwitch : DareLib/Dare/getAPI_type  g_funcname=Rte_GetVfb_DrHeightSwitchCmd  g_param=""  g_type=uint8  g_size=-1
      settings: AttributesFormatString=%<g_funcname>  SourceProductName=Dare Library
  DrMem_IVI_FLSeatMemSet1 : DareLib/Dare/getAPI_type  g_funcname=CanRx_0x351_IVI_FLSeatMemSet1  g_param=""  g_type=uint8  g_enum=enMemSet  g_size=-1
      settings: AttributesFormatString=%<g_funcname>  SourceProductName=Dare Library
  DrMem_IVI_FLSeatMemSet2 : DareLib/Dare/getAPI_type  g_funcname=CanRx_0x351_IVI_FLSeatMemSet2  g_param=""  g_type=uint8  g_enum=enMemSet  g_size=-1
      settings: AttributesFormatString=%<g_funcname>  SourceProductName=Dare Library
  DrMem_IVI_FLSeatMemSet3 : DareLib/Dare/getAPI_type  g_funcname=CanRx_0x351_IVI_FLSeatMemSet3  g_param=""  g_type=uint8  g_enum=enMemSet  g_size=-1
      settings: AttributesFormatString=%<g_funcname>  SourceProductName=Dare Library
  DrMem_LengthAutoRunFlag : DareLib/Dare/getAPI_type  g_funcname=Rte_GetVfb_DrLengthAutoRunFlag  g_param=""  g_type=uint8  g_enum=enSeatAutoRunSts  g_size=-1
      settings: AttributesFormatString=%<g_funcname>  SourceProductName=Dare Library
  DrMem_LengthHallPosi : DareLib/Dare/getAPI_type  g_funcname=Cdd_GetCurrentHallCnt  g_param=EN_DriverLength  g_type=uint16  g_size=-1
      settings: AttributesFormatString=%<g_funcname>  SourceProductName=Dare Library
  DrMem_LengthLockFault : DareLib/Dare/getAPI_type  g_funcname=Rte_GetVfb_DrLengthStallErr  g_param=""  g_type=uint8  g_size=-1
      settings: AttributesFormatString=%<g_funcname>  SourceProductName=Dare Library
  DrMem_LengthMem1 : DareLib/Dare/getAPI_type  g_funcname=Srvl_GetMemIndexDataU16  g_param=EN_MemIndex_DrMem1_Length  g_type=uint16  g_size=-1
      settings: AttributesFormatString=%<g_funcname>  SourceProductName=Dare Library
  DrMem_LengthMem2 : DareLib/Dare/getAPI_type  g_funcname=Srvl_GetMemIndexDataU16  g_param=EN_MemIndex_DrMem2_Length  g_type=uint16  g_size=-1
      settings: AttributesFormatString=%<g_funcname>  SourceProductName=Dare Library
  DrMem_LengthMem3 : DareLib/Dare/getAPI_type  g_funcname=Srvl_GetMemIndexDataU16  g_param=EN_MemIndex_DrMem3_Length  g_type=uint16  g_size=-1
      settings: AttributesFormatString=%<g_funcname>  SourceProductName=Dare Library
  DrMem_LengthSwitch : DareLib/Dare/getAPI_type  g_funcname=Rte_GetVfb_DrLengthSwitchCmd  g_param=""  g_type=uint8  g_size=-1
      settings: AttributesFormatString=%<g_funcname>  SourceProductName=Dare Library
  DrMem_MemoryConfig : DareLib/Dare/getAPI_type  g_funcname=Srvl_GetMemIndexDataU8  g_param=EN_MemIndex_DrMemoryConfig  g_type=uint8  g_size=-1
      settings: AttributesFormatString=%<g_funcname>  SourceProductName=Dare Library
  DrMem_NapMode : DareLib/Dare/getAPI_type  g_funcname=Rte_GetVfb_NapMode  g_param=""  g_type=uint8  g_enum=enNapMode  g_size=-1
      settings: AttributesFormatString=%<g_funcname>  SourceProductName=Dare Library
  DrMem_PowerMode : DareLib/Dare/getAPI_type  g_funcname=Rte_GetVfb_PowerMode  g_param=""  g_type=uint8  g_enum=enPowerModeSts  g_size=-1
      settings: AttributesFormatString=%<g_funcname>  SourceProductName=Dare Library
  DrMem_SeatLearnResult : DareLib/Dare/getAPI_type  g_funcname=Rte_GetVfb_DrLearnResult  g_param=""  g_type=uint8  g_size=-1
      settings: AttributesFormatString=%<g_funcname>  SourceProductName=Dare Library
  DrMem_SeatMemory1Valid : DareLib/Dare/getAPI_type  g_funcname=Srvl_GetMemIndexDataU8  g_param=EN_MemIndex_DrMem1_ValidFlag  g_type=uint8  g_size=-1
      settings: AttributesFormatString=%<g_funcname>  SourceProductName=Dare Library
  DrMem_SeatMemory2Valid : DareLib/Dare/getAPI_type  g_funcname=Srvl_GetMemIndexDataU8  g_param=EN_MemIndex_DrMem2_ValidFlag  g_type=uint8  g_size=-1
      settings: AttributesFormatString=%<g_funcname>  SourceProductName=Dare Library
  DrMem_SeatMemory3Valid : DareLib/Dare/getAPI_type  g_funcname=Srvl_GetMemIndexDataU8  g_param=EN_MemIndex_DrMem3_ValidFlag  g_type=uint8  g_size=-1
      settings: AttributesFormatString=%<g_funcname>  SourceProductName=Dare Library
  DrMem_VehicleSpeed : DareLib/Dare/getAPI_type  g_funcname=CanRx_0x284_ABS_VehicleSpeed  g_param=""  g_type=uint16  g_size=-1
      settings: AttributesFormatString=%<g_funcname>  SourceProductName=Dare Library
  DrMem_VehicleSpeedValid : DareLib/Dare/getAPI_type  g_funcname=CanRx_0x284_ABS_VehicleSpeedValid  g_param=""  g_type=uint8  g_size=-1
      settings: AttributesFormatString=%<g_funcname>  SourceProductName=Dare Library
  DrMem_VoltMode : DareLib/Dare/getAPI_type  g_funcname=Rte_GetVfb_VoltMode  g_param=""  g_type=uint8  g_enum=enFinalPowerMode  g_size=-1
      settings: AttributesFormatString=%<g_funcname>  SourceProductName=Dare Library
  DrMem_VoltSatisfy : DareLib/Dare/getAPI_type  g_funcname=Rte_GetVfb_VoltSatisfy  g_param=""  g_type=uint8  g_size=-1
      settings: AttributesFormatString=%<g_funcname>  SourceProductName=Dare Library
  RTE_Signal : Outport
  wires:
  Bus Creator/1 -> RTE_Signal/1  "RTE_Signal"
  DrMem_HeightSwitch/1 -> Bus Creator/1  "DrMem_HeightSwitch"
  DrMem_LengthSwitch/1 -> Bus Creator/2  "DrMem_LengthSwitch"
  DrMem_BackSwitch/1 -> Bus Creator/3  "DrMem_BackSwitch"
  DrMem_FrontSwitch/1 -> Bus Creator/4  "DrMem_FrontSwitch"
  DrMem_HeightAutoRunFlag/1 -> Bus Creator/5  "DrMem_HeightAutoRunFlag"
  DrMem_LengthAutoRunFlag/1 -> Bus Creator/6  "DrMem_LengthAutoRunFlag"
  DrMem_BackAutoRunFlag/1 -> Bus Creator/7  "DrMem_BackAutoRunFlag"
  DrMem_FrontAutoRunFlag/1 -> Bus Creator/8  "DrMem_FrontAutoRunFlag"
  DrMem_HeightLockFault/1 -> Bus Creator/9  "DrMem_HeightLockFault"
  DrMem_LengthLockFault/1 -> Bus Creator/10  "DrMem_LengthLockFault"
  DrMem_BackLockFault/1 -> Bus Creator/11  "DrMem_BackLockFault"
  DrMem_FrontLockFault/1 -> Bus Creator/12  "DrMem_FrontLockFault"
  DrMem_DtcAnyoneHallFaultSts/1 -> Bus Creator/13  "DrMem_DtcAnyoneHallFaultSts"
  DrMem_AnyoneRelayFaultSts/1 -> Bus Creator/14  "DrMem_AnyoneRelayFaultSts"
  DrMem_AnyoneLockFaultSts/1 -> Bus Creator/15  "DrMem_AnyoneLockFaultSts"
  DrMem_Gear_PN_FlagOut/1 -> Bus Creator/16  "DrMem_Gear_PN_FlagOut"
  DrMem_CurrentMoveType/1 -> Bus Creator/17  "DrMem_CurrentMoveType"
  DrMem_HeightHallPosi/1 -> Bus Creator/18  "DrMem_HeightHallPosi"
  DrMem_LengthHallPosi/1 -> Bus Creator/19  "DrMem_LengthHallPosi"
  DrMem_BackHallPosi/1 -> Bus Creator/20  "DrMem_BackHallPosi"
  DrMem_FrontHallPosi/1 -> Bus Creator/21  "DrMem_FrontHallPosi"
  DrMem_HeightMem1/1 -> Bus Creator/22  "DrMem_HeightMem1"
  DrMem_LengthMem1/1 -> Bus Creator/23  "DrMem_LengthMem1"
  DrMem_BackMem1/1 -> Bus Creator/24  "DrMem_BackMem1"
  DrMem_FrontMem1/1 -> Bus Creator/25  "DrMem_FrontMem1"
  DrMem_HeightMem2/1 -> Bus Creator/26  "DrMem_HeightMem2"
  DrMem_LengthMem2/1 -> Bus Creator/27  "DrMem_LengthMem2"
  DrMem_BackMem2/1 -> Bus Creator/28  "DrMem_BackMem2"
  DrMem_FrontMem2/1 -> Bus Creator/29  "DrMem_FrontMem2"
  DrMem_HeightMem3/1 -> Bus Creator/30  "DrMem_HeightMem3"
  DrMem_LengthMem3/1 -> Bus Creator/31  "DrMem_LengthMem3"
  DrMem_BackMem3/1 -> Bus Creator/32  "DrMem_BackMem3"
  DrMem_FrontMem3/1 -> Bus Creator/33  "DrMem_FrontMem3"
  DrMem_FLSeatPosMsg/1 -> Bus Creator/34  "DrMem_FLSeatPosMsg"
  DrMem_AdjustEnable/1 -> Bus Creator/35  "DrMem_AdjustEnable"
  DrMem_VehicleSpeed/1 -> Bus Creator/36  "DrMem_VehicleSpeed"
  DrMem_VehicleSpeedValid/1 -> Bus Creator/37  "DrMem_VehicleSpeedValid"
  DrMem_IVI_FLSeatMemSet1/1 -> Bus Creator/38  "DrMem_IVI_FLSeatMemSet1"
  DrMem_IVI_FLSeatMemSet2/1 -> Bus Creator/39  "DrMem_IVI_FLSeatMemSet2"
  DrMem_IVI_FLSeatMemSet3/1 -> Bus Creator/40  "DrMem_IVI_FLSeatMemSet3"
  DrMem_SeatMemory1Valid/1 -> Bus Creator/41  "DrMem_SeatMemory1Valid"
  DrMem_SeatMemory2Valid/1 -> Bus Creator/42  "DrMem_SeatMemory2Valid"
  DrMem_SeatMemory3Valid/1 -> Bus Creator/43  "DrMem_SeatMemory3Valid"
  DrMem_SeatLearnResult/1 -> Bus Creator/44  "DrMem_SeatLearnResult"
  DrMem_GetRecoverDefaultFlag/1 -> Bus Creator/45  "DrMem_GetRecoverDefaultFlag"
  DrMem_NapMode/1 -> Bus Creator/46  "DrMem_NapMode"
  DrMem_MemoryConfig/1 -> Bus Creator/47  "DrMem_MemoryConfig"
  DrMem_PowerMode/1 -> Bus Creator/48  "DrMem_PowerMode"
  DrMem_VoltMode/1 -> Bus Creator/49  "DrMem_VoltMode"
  DrMem_VoltSatisfy/1 -> Bus Creator/50  "DrMem_VoltSatisfy"
  DrMem_0x284_SpeedLostFlag/1 -> Bus Creator/51  "DrMem_0x284_SpeedLostFlag"

== system Appl_DrMemory_CtrlModel/LogicCtrl/LocalAdjustCtrl/MemoryCall/GetCanSendEvent ==
  f : TriggerPort  TriggerType=function-call  VariantControl=(inherit)
      settings: CopyFcn=Stateflow.SLINSF.SimulinkMan.removeBlockPreDeleteFcn  PreDeleteFcn=Stateflow.SLINSF.SimulinkMan.unsafePredeleteFcn
  DrMem_FrontHallPosi : DareLib/Dare/getAPI_type  g_funcname=Rte_GetCanEventSendTimes_0x3B2  g_param=""  g_type=uint16  g_size=-1
      settings: AttributesFormatString=%<g_funcname>  SourceProductName=Dare Library
  Out1 : Outport
  wires:
  DrMem_FrontHallPosi/1 -> Out1/1

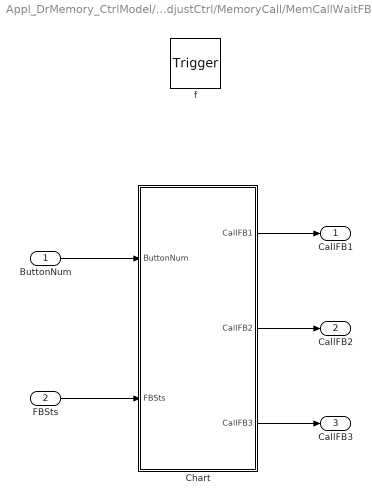
== system Appl_DrMemory_CtrlModel/LogicCtrl/LocalAdjustCtrl/MemoryCall/MemCallWaitFBFunc ==
  ButtonNum : Inport
  FBSts : Inport  Port=2
  f : TriggerPort  TriggerType=function-call  VariantControl=(inherit)
      settings: CopyFcn=Stateflow.SLINSF.SimulinkMan.removeBlockPreDeleteFcn  PreDeleteFcn=Stateflow.SLINSF.SimulinkMan.unsafePredeleteFcn
  Chart : Stateflow chart  TreatAsAtomicUnit=on
  CallFB1 : Outport
  CallFB2 : Outport  Port=2
  CallFB3 : Outport  Port=3
  wires:
  ButtonNum/1 -> Chart/1(ButtonNum)
  FBSts/1 -> Chart/2(FBSts)
  Chart/1(CallFB1) -> CallFB1/1
  Chart/2(CallFB2) -> CallFB2/1
  Chart/3(CallFB3) -> CallFB3/1

== system Appl_DrMemory_CtrlModel/LogicCtrl/LocalAdjustCtrl/MemoryCall/SetCanMemCall1 ==
  In1 : Inport
  f : TriggerPort  TriggerType=function-call  VariantControl=(inherit)
      settings: CopyFcn=Stateflow.SLINSF.SimulinkMan.removeBlockPreDeleteFcn  PreDeleteFcn=Stateflow.SLINSF.SimulinkMan.unsafePredeleteFcn
  DrMemO_SeatMem1StsFb : DareLib/Dare/setAPI_type  g_funcname=CanTx_0x3B2_DSM1_FLSeatMem1Sts  g_param=""  g_type=uint16  g_size=-1
      settings: AttributesFormatString=%<g_funcname>  SourceProductName=Dare Library
  wires:
  In1/1 -> DrMemO_SeatMem1StsFb/1

== system Appl_DrMemory_CtrlModel/LogicCtrl/LocalAdjustCtrl/MemoryCall/SetCanMemCall2 ==
  In1 : Inport
  f : TriggerPort  TriggerType=function-call  VariantControl=(inherit)
      settings: CopyFcn=Stateflow.SLINSF.SimulinkMan.removeBlockPreDeleteFcn  PreDeleteFcn=Stateflow.SLINSF.SimulinkMan.unsafePredeleteFcn
  DrMemO_SeatMem1StsFb : DareLib/Dare/setAPI_type  g_funcname=CanTx_0x3B2_DSM2_FLSeatMem2Sts  g_param=""  g_type=uint16  g_size=-1
      settings: AttributesFormatString=%<g_funcname>  SourceProductName=Dare Library
  wires:
  In1/1 -> DrMemO_SeatMem1StsFb/1

== system Appl_DrMemory_CtrlModel/LogicCtrl/LocalAdjustCtrl/MemoryCall/SetCanMemCall3 ==
  In1 : Inport
  f : TriggerPort  TriggerType=function-call  VariantControl=(inherit)
      settings: CopyFcn=Stateflow.SLINSF.SimulinkMan.removeBlockPreDeleteFcn  PreDeleteFcn=Stateflow.SLINSF.SimulinkMan.unsafePredeleteFcn
  DrMemO_SeatMem1StsFb : DareLib/Dare/setAPI_type  g_funcname=CanTx_0x3B2_DSM3_FLSeatMem3Sts  g_param=""  g_type=uint16  g_size=-1
      settings: AttributesFormatString=%<g_funcname>  SourceProductName=Dare Library
  wires:
  In1/1 -> DrMemO_SeatMem1StsFb/1

== system Appl_DrMemory_CtrlModel/LogicCtrl/LocalAdjustCtrl/MemoryCall/SetCanSendEvent ==
  f : TriggerPort  TriggerType=function-call  VariantControl=(inherit)
      settings: CopyFcn=Stateflow.SLINSF.SimulinkMan.removeBlockPreDeleteFcn  PreDeleteFcn=Stateflow.SLINSF.SimulinkMan.unsafePredeleteFcn
  DrMemO_SeatMem1StsFb : DareLib/Dare/setAPI_type  g_funcname=Rte_SetCanEvent_0x3B2  g_param=""  g_type=uint16  g_size=-1
      settings: AttributesFormatString=%<g_funcname>  SourceProductName=Dare Library

== system Appl_DrMemory_CtrlModel/LogicCtrl/LocalAdjustCtrl/MemoryRemindLogic/GetCanSendEvent ==
  f : TriggerPort  TriggerType=function-call  VariantControl=(inherit)
      settings: CopyFcn=Stateflow.SLINSF.SimulinkMan.removeBlockPreDeleteFcn  PreDeleteFcn=Stateflow.SLINSF.SimulinkMan.unsafePredeleteFcn
  DrMem_FrontHallPosi : DareLib/Dare/getAPI_type  g_funcname=Rte_GetCanEventSendTimes_0x3B2  g_param=""  g_type=uint16  g_size=-1
      settings: AttributesFormatString=%<g_funcname>  SourceProductName=Dare Library
  Out1 : Outport
  wires:
  DrMem_FrontHallPosi/1 -> Out1/1

== system Appl_DrMemory_CtrlModel/LogicCtrl/LocalAdjustCtrl/MemoryRemindLogic/SetCanSendEvent ==
  f : TriggerPort  TriggerType=function-call  VariantControl=(inherit)
      settings: CopyFcn=Stateflow.SLINSF.SimulinkMan.removeBlockPreDeleteFcn  PreDeleteFcn=Stateflow.SLINSF.SimulinkMan.unsafePredeleteFcn
  DrMemO_SeatMem1StsFb : DareLib/Dare/setAPI_type  g_funcname=Rte_SetCanEvent_0x3B2  g_param=""  g_type=uint16  g_size=-1
      settings: AttributesFormatString=%<g_funcname>  SourceProductName=Dare Library

== system Appl_DrMemory_CtrlModel/LogicCtrl/LocalAdjustCtrl/MemoryRemindLogic/SetCanSendFLSeatPosMsg ==
  In1 : Inport
  f : TriggerPort  TriggerType=function-call  VariantControl=(inherit)
      settings: CopyFcn=Stateflow.SLINSF.SimulinkMan.removeBlockPreDeleteFcn  PreDeleteFcn=Stateflow.SLINSF.SimulinkMan.unsafePredeleteFcn
  DrMemO_SeatMem1StsFb : DareLib/Dare/setAPI_type  g_funcname=CanTx_0x3B2_DSM_FLSeatPosMsg  g_param=""  g_type=uint16  g_size=-1
      settings: AttributesFormatString=%<g_funcname>  SourceProductName=Dare Library
  wires:
  In1/1 -> DrMemO_SeatMem1StsFb/1

== system Appl_DrMemory_CtrlModel/LogicCtrl/LocalAdjustCtrl/MemoryRemindLogic/WriteFLSeatPosMsg ==
  Sts : Inport
  f : TriggerPort  TriggerType=function-call  VariantControl=(inherit)
      settings: CopyFcn=Stateflow.SLINSF.SimulinkMan.removeBlockPreDeleteFcn  PreDeleteFcn=Stateflow.SLINSF.SimulinkMan.unsafePredeleteFcn
  DrMemO_SeatBackPosiReq : DareLib/Dare/setAPI_type  g_funcname=Srvl_SetMemIndexDataU8  g_param=EN_MemIndex_FLSeatPosMsg  g_type=uint16  g_size=-1
      settings: AttributesFormatString=%<g_funcname>  SourceProductName=Dare Library
  wires:
  Sts/1 -> DrMemO_SeatBackPosiReq/1

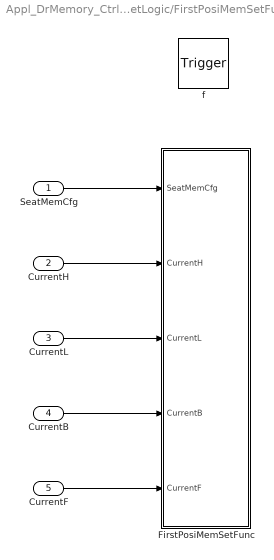
== system Appl_DrMemory_CtrlModel/LogicCtrl/LocalAdjustCtrl/MemorySetLogic/FirstPosiMemSetFunc ==
  SeatMemCfg : Inport
  CurrentH : Inport  Port=2
  CurrentL : Inport  Port=3
  CurrentB : Inport  Port=4
  CurrentF : Inport  Port=5
  f : TriggerPort  TriggerType=function-call  VariantControl=(inherit)
      settings: CopyFcn=Stateflow.SLINSF.SimulinkMan.removeBlockPreDeleteFcn  PreDeleteFcn=Stateflow.SLINSF.SimulinkMan.unsafePredeleteFcn
  FirstPosiMemSetFunc : Stateflow chart  TreatAsAtomicUnit=on
  wires:
  CurrentH/1 -> FirstPosiMemSetFunc/2(CurrentH)
  CurrentL/1 -> FirstPosiMemSetFunc/3(CurrentL)
  SeatMemCfg/1 -> FirstPosiMemSetFunc/1(SeatMemCfg)
  CurrentB/1 -> FirstPosiMemSetFunc/4(CurrentB)
  CurrentF/1 -> FirstPosiMemSetFunc/5(CurrentF)

== system Appl_DrMemory_CtrlModel/LogicCtrl/LocalAdjustCtrl/MemorySetLogic/GetCanSendEvent ==
  f : TriggerPort  TriggerType=function-call  VariantControl=(inherit)
      settings: CopyFcn=Stateflow.SLINSF.SimulinkMan.removeBlockPreDeleteFcn  PreDeleteFcn=Stateflow.SLINSF.SimulinkMan.unsafePredeleteFcn
  DrMem_FrontHallPosi : DareLib/Dare/getAPI_type  g_funcname=Rte_GetCanEventSendTimes_0x3B2  g_param=""  g_type=uint8  g_size=-1
      settings: AttributesFormatString=%<g_funcname>  SourceProductName=Dare Library
  Out1 : Outport
  wires:
  DrMem_FrontHallPosi/1 -> Out1/1

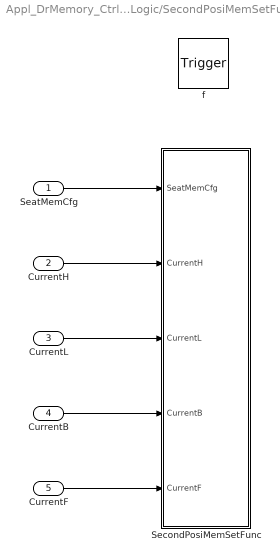
== system Appl_DrMemory_CtrlModel/LogicCtrl/LocalAdjustCtrl/MemorySetLogic/SecondPosiMemSetFunc ==
  SeatMemCfg : Inport
  CurrentH : Inport  Port=2
  CurrentL : Inport  Port=3
  CurrentB : Inport  Port=4
  CurrentF : Inport  Port=5
  f : TriggerPort  TriggerType=function-call  VariantControl=(inherit)
      settings: CopyFcn=Stateflow.SLINSF.SimulinkMan.removeBlockPreDeleteFcn  PreDeleteFcn=Stateflow.SLINSF.SimulinkMan.unsafePredeleteFcn
  SecondPosiMemSetFunc : Stateflow chart  TreatAsAtomicUnit=on
  wires:
  CurrentH/1 -> SecondPosiMemSetFunc/2(CurrentH)
  CurrentL/1 -> SecondPosiMemSetFunc/3(CurrentL)
  SeatMemCfg/1 -> SecondPosiMemSetFunc/1(SeatMemCfg)
  CurrentB/1 -> SecondPosiMemSetFunc/4(CurrentB)
  CurrentF/1 -> SecondPosiMemSetFunc/5(CurrentF)

== system Appl_DrMemory_CtrlModel/LogicCtrl/LocalAdjustCtrl/MemorySetLogic/SetCanSendEvent ==
  f : TriggerPort  TriggerType=function-call  VariantControl=(inherit)
      settings: CopyFcn=Stateflow.SLINSF.SimulinkMan.removeBlockPreDeleteFcn  PreDeleteFcn=Stateflow.SLINSF.SimulinkMan.unsafePredeleteFcn
  DrMemO_SeatMem1StsFb : DareLib/Dare/setAPI_type  g_funcname=Rte_SetCanEvent_0x3B2  g_param=""  g_type=uint16  g_size=-1
      settings: AttributesFormatString=%<g_funcname>  SourceProductName=Dare Library

== system Appl_DrMemory_CtrlModel/LogicCtrl/LocalAdjustCtrl/MemorySetLogic/SetCanSendFLSeatMemSts ==
  In1 : Inport
  f : TriggerPort  TriggerType=function-call  VariantControl=(inherit)
      settings: CopyFcn=Stateflow.SLINSF.SimulinkMan.removeBlockPreDeleteFcn  PreDeleteFcn=Stateflow.SLINSF.SimulinkMan.unsafePredeleteFcn
  DrMemO_SeatMem1StsFb : DareLib/Dare/setAPI_type  g_funcname=CanTx_0x3B2_DSM_FLSeatMemStsAndMsg  g_param=""  g_type=uint16  g_size=-1
      settings: AttributesFormatString=%<g_funcname>  SourceProductName=Dare Library
  wires:
  In1/1 -> DrMemO_SeatMem1StsFb/1

== system Appl_DrMemory_CtrlModel/LogicCtrl/LocalAdjustCtrl/MemorySetLogic/ThirdPosiMemSetFunc ==
  SeatMemCfg : Inport
  CurrentH : Inport  Port=2
  CurrentL : Inport  Port=3
  CurrentB : Inport  Port=4
  CurrentF : Inport  Port=5
  f : TriggerPort  TriggerType=function-call  VariantControl=(inherit)
      settings: CopyFcn=Stateflow.SLINSF.SimulinkMan.removeBlockPreDeleteFcn  PreDeleteFcn=Stateflow.SLINSF.SimulinkMan.unsafePredeleteFcn
  ThirdPosiMemSetFunc : Stateflow chart  TreatAsAtomicUnit=on
  wires:
  CurrentH/1 -> ThirdPosiMemSetFunc/2(CurrentH)
  CurrentL/1 -> ThirdPosiMemSetFunc/3(CurrentL)
  SeatMemCfg/1 -> ThirdPosiMemSetFunc/1(SeatMemCfg)
  CurrentB/1 -> ThirdPosiMemSetFunc/4(CurrentB)
  CurrentF/1 -> ThirdPosiMemSetFunc/5(CurrentF)
